simulink model "fuzzyFinalPDI"  (R2020b)
settings: Solver=VariableStepAuto  StartTime=0.0  StopTime=100  RelTol=1e-3
libraries: fuzblock x1
settings Model: Creator=Daniela  LastModifiedBy=Daniela

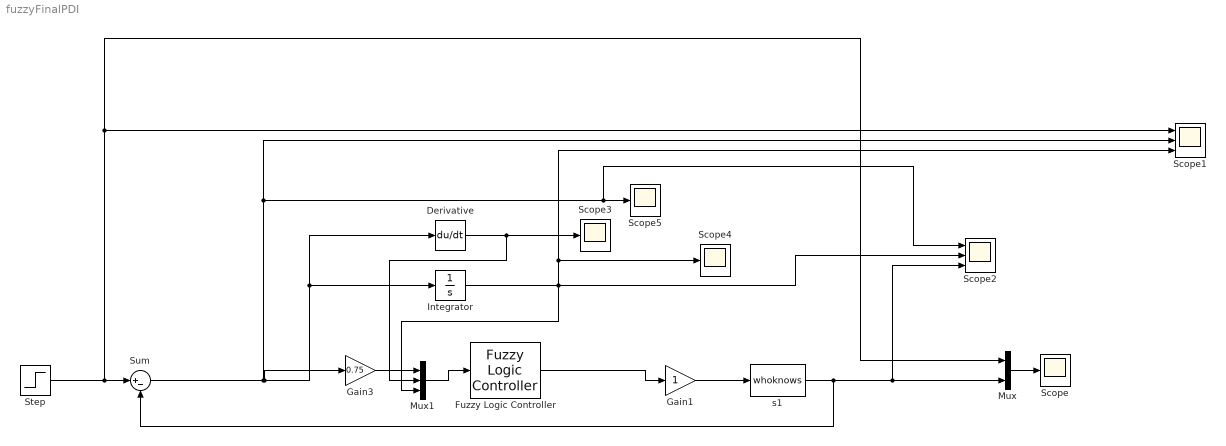
== system fuzzyFinalPDI ==
  Derivative : Derivative
  Fuzzy Logic Controller : fuzblock/Fuzzy Logic  Controller  FIS='FuzzyPDI_Final.fis'  OutputSampleNumber=101  DataType=double  FuzzifiedInputs=off  RuleFiringStrengths=off  RuleOutputs=off  AggregatedOutputs=off  SimulateUsing=Interpreted execution  OutOfRangeInputValueMessage=warning  NoRuleFiredMessage=warning  EmptyOutputFuzzySetMessage=warning
  Gain1 : Gain
  Gain3 : Gain  Gain=0.75
  Integrator : Integrator
  Mux : Mux  Inputs=2
  Mux1 : Mux  Inputs=3
  Scope{,3..5} (4 alike) : Scope
  Scope1 : Scope  NumInputPorts=3
  Scope2 : Scope  NumInputPorts=3
  Step : Step  SampleTime=0
  Sum : Sum  Inputs=|+-
  s1 : M-S-Function  FunctionName=whoknows  Parameters=L, P1, P2, T, R  mask{L=7, P1=0, P2=7, T=2, R=0}
      mask prompts: L "Laboratorio"; P1 "Primer digito del Puesto"; P2 "Segundo digito del Puesto"; T "Tipo de Planta"; R "Ruido"
      mask Display: disp('Sistema')
  wires:
  Fuzzy Logic Controller/1 -> Gain1/1
  Integrator/1 -> Scope2/2, Scope4/1, Scope1/3, Mux1/3
  Derivative/1 -> Mux1/2, Scope3/1
  Mux1/1 -> Fuzzy Logic Controller/1
  Step/1 -> Sum/1, Scope1/1, Mux/1
  s1/1 -> Scope2/3, Mux/2, Sum/2
  Gain1/1 -> s1/1
  Sum/1 -> Gain3/1, Integrator/1, Derivative/1, Scope2/1, Scope5/1, Scope1/2
  Mux/1 -> Scope/1
  Gain3/1 -> Mux1/1
